simulink model "testmodel"  (R2021a)
settings: Solver=VariableStepAuto  StartTime=0.0  StopTime=10.0  RelTol=1e-3
undefined symbols (not defined in the file): B, K, M
settings Model: Creator=MC2  LastModifiedBy=MC2

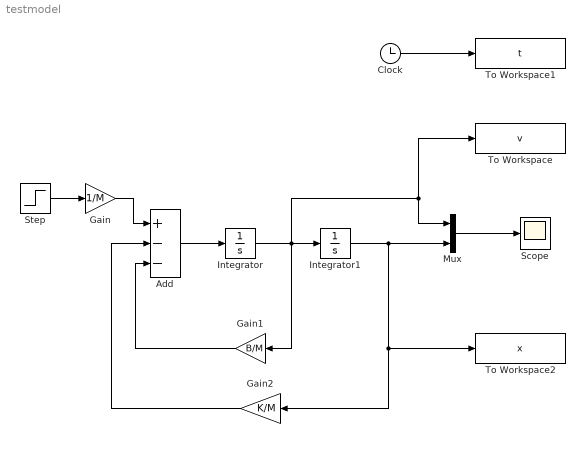
== system testmodel ==
  Add : Sum  Inputs=+--
  Clock : Clock
  Gain : Gain  Gain=1/M
  Gain1 : Gain  Gain=B/M
  Gain2 : Gain  Gain=K/M
  Integrator : Integrator
  Integrator1 : Integrator
  Mux : Mux  Inputs=2
  Scope : Scope
  Step : Step  After=8  SampleTime=0
  To Workspace : ToWorkspace  VariableName=v  SampleTime=-1
  To Workspace1 : ToWorkspace  VariableName=t  SampleTime=-1
  To Workspace2 : ToWorkspace  VariableName=x  SampleTime=-1
  wires:
  Step/1 -> Gain/1
  Add/1 -> Integrator/1
  Integrator/1 -> Gain1/1, Mux/1, To Workspace/1, Integrator1/1
  Integrator1/1 -> To Workspace2/1, Gain2/1, Mux/2
  Mux/1 -> Scope/1
  Clock/1 -> To Workspace1/1
  Gain/1 -> Add/1
  Gain1/1 -> Add/3
  Gain2/1 -> Add/2
